simulink model "lab1template2"  (R2018a)
settings: Solver=FixedStepDiscrete  StartTime=0.0  StopTime=17.97  FixedStep=0.03  RelTol=1e-3  EnableMultiTasking=on
libraries: simulink x2, MinSegLibrary_M1V4 x2
settings Model: SimulationMode=external  ExtModeTrigDuration=2  Creator=Magnus  LastModifiedBy=Magnus
settings OptimizationCC: EnhancedBackFolding=on  PassReuseOutputArgsThreshold=0  MaxStackSize=64  OptimizeBlockOrder=speed  DifferentSizesBufferReuse=on  OptimizationCustomize=off
settings DebuggingCC: ParameterTunabilityLossMsg=error
settings HardwareCC: ProdBitPerInt=16  ProdBitPerPointer=16  ProdBitPerSizeT=16  ProdBitPerPtrDiffT=16  ProdLargestAtomicFloat=None  ProdWordSize=8  ProdHWDeviceType=Atmel->AVR  UseEmbeddedCoderFeatures=off  UseSimulinkCoderFeatures=off
settings SFSimCC: MATLABDynamicMemAlloc=off
settings RTWCC: SystemTargetFile=ert.tlc  HardwareBoard=Arduino Mega 2560  TLCOptions=-aInlineSetEventsForThisBaseRateFcn=TLC_FALSE -aSuppressMultiTaskScheduler=TLC_FALSE -aRateBasedStepFcn=1  TemplateMakefile=ert_default_tmf  GenerateReport=on  Toolchain=Arduino AVR  BuildConfiguration=Faster Runs  LaunchReport=on
settings CodeAppCC: ForceParamTrailComments=on  OperatorAnnotations=on
settings ERTTargetCC: ERTCustomFileBanners=off  SupportContinuousTime=on  SupportNonInlinedSFcns=on  RemoveResetFunc=off  SupportVariableSizeSignals=on  ModelStepFunctionPrototypeControlCompliant=off

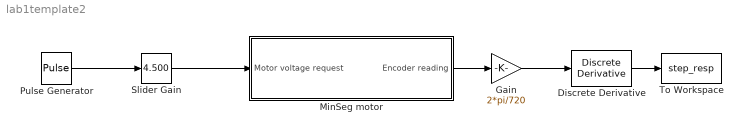
== system lab1template2 ==
  Discrete Derivative : simulink/Discrete/Discrete Derivative  gainval=1.0  ICPrevScaledInput=0.0  OutMin=[]  OutMax=[]  OutDataTypeStr=double  OutputDataTypeScalingMode=double  OutDataType=fixdt(1, 16)  OutScaling=2^-10  DoSatur=off
  Gain : Gain  Gain=2*pi/720
  MinSeg motor : Subsystem
  Pulse Generator : DiscretePulseGenerator  Period=60  PulseWidth=35  SampleTime=-1
  Slider Gain : simulink/Math Operations/Slider Gain  gain=4.500  low=0  high=4.5
  To Workspace : ToWorkspace  VariableName=step_resp  SampleTime=-1
  wires:
  Pulse Generator/1 -> Slider Gain/1
  Slider Gain/1 -> MinSeg motor/1(Motor voltage request)
  MinSeg motor/1(Encoder reading) -> Gain/1
  Discrete Derivative/1 -> To Workspace/1
  Gain/1 -> Discrete Derivative/1

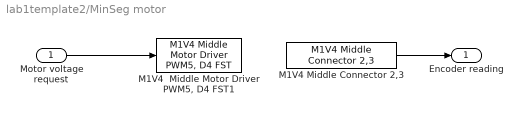
== system lab1template2/MinSeg motor ==
  Motor voltage request : Inport
  "M1V4  Middle Motor Driver PWM5, D4 FST1" : MinSegLibrary_M1V4/M1V4  Middle Motor Driver PWM5, D4 FST  Vsupply=4.5
      settings: SourceProductName=Rensselaer Arduino Support Package
  M1V4 Middle Connector 2,3 : MinSegLibrary_M1V4/M1V4 Middle Connector 2,3  Encoder=0  PinA=3  PinB=2
      settings: SourceProductName=Rensselaer Arduino Support Package
  Encoder reading : Outport
  wires:
  M1V4 Middle Connector 2,3/1 -> Encoder reading/1
  Motor voltage request/1 -> "M1V4  Middle Motor Driver PWM5, D4 FST1"/1
